simulink model "PWM_PI_PE_2018b"  (R2018b)
settings: Solver=VariableStepAuto  StartTime=0.0  StopTime=10e-3  RelTol=1e-3
values from neighbouring files (symbols this model uses):
  Ap = wc*Tr    (= 0.861890988639)    [PWM_szab_init.m]
  fs = 20e3    (= 20000)    [PWM_szab_init.m]
  k_peak = 10    [PWM_szab_init.m]
  Ki = xref_n/Iki_n    (= 1)    [PWM_szab_init.m]
  R = 0.1    [PWM_szab_init.m]
  tau_Ki = 2e-6    (= 2e-06)    [PWM_szab_init.m]
  TI = 1/(wc*tan((pi/2-fi_t)*1/3))    [PWM_szab_init.m]
undefined symbols (not defined in the file or in its folder): sigbuilder_block
libraries: ee_lib x8, nesl_utility x6, fl_lib x4, simulink x1
settings Model: Creator=kissd  LastModifiedBy=kissd
settings DataIOCC: ReturnWorkspaceOutputs=on

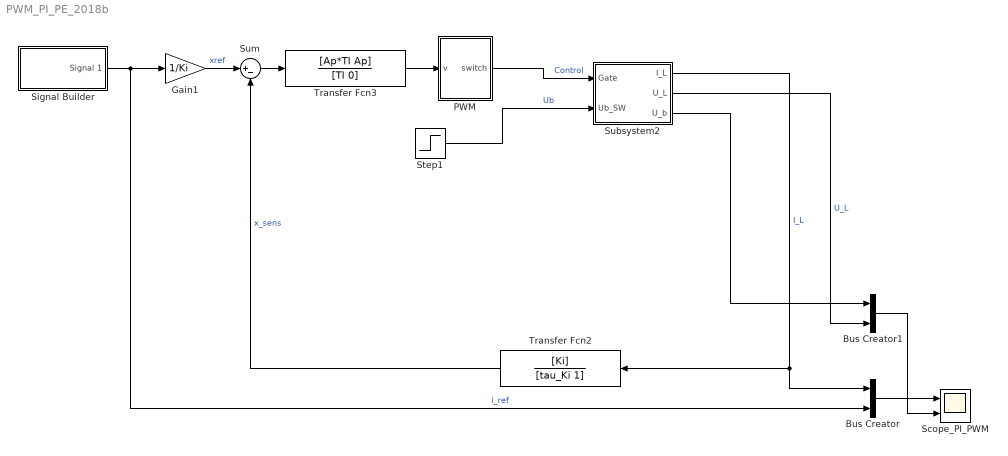
== system PWM_PI_PE_2018b ==
  Bus Creator : BusCreator  Inputs=2
  Bus Creator1 : BusCreator  Inputs=2
  Gain1 : Gain  Gain=1/Ki
  PWM : Subsystem
  Scope_PI_PWM : Scope  NumInputPorts=2
  Signal Builder : Subsystem  Tag=STV Subsys  LoadFcn=sigbuilder_block('load');  StartFcn=sigbuilder_block('start');  StopFcn=sigbuilder_block('stop');  ClipboardFcn=sigbuilder_block('clipboard');  mask(Sigbuilder block){tuvar=[0:10]}
      mask help: Simulink:masks:SigbuilderBlock_MD
      mask init:
      | if ~strcmp(get_param(bdroot(gcbh),'SimulationStatus'),'stopped') tuvar = sigbuilder_block('maskInit'); end
      settings: CopyFcn=sigbuilder_block('copy');  DeleteFcn=sigbuilder_block('delete');  ModelCloseFcn=sigbuilder_block('modelClose');  PreSaveFcn=sigbuilder_block('preSave');  PauseFcn=sigbuilder_block('pause');  ContinueFcn=sigbuilder_block('continue');  NameChangeFcn=sigbuilder_block('namechange');  OpenFcn=sigbuilder_block('open',[437.25 118.5 550.5 394.5 ]);  CloseFcn=sigbuilder_block('close');
      mask Display: plot(0, 0, 100, 100,[2, 2, 32, 32, 2], [68, 8, 8, 68, 68],[32, 2], [38, 38], [32, 19, 2],[53, 60, 44], [32, 17, 17, 2],[16, 16, 31, 31]);txt = getActiveGroup(gcbh);text(2, 100, txt,'verticalAlignment', 'top');
  Step1 : Step  Time=6e-3  SampleTime=0
  Subsystem2 : Subsystem
  Sum : Sum  Inputs=|+-
  Transfer Fcn2 : TransferFcn  Numerator=[Ki]  Denominator=[tau_Ki 1]
  Transfer Fcn3 : TransferFcn  Numerator=[Ap*TI Ap]  Denominator=[TI 0]
  wires:
  Transfer Fcn3/1 -> PWM/1(v)
  Signal Builder/1(Signal 1) -> Bus Creator/2, Gain1/1  "i_ref"
  Bus Creator/1 -> Scope_PI_PWM/1
  Bus Creator1/1 -> Scope_PI_PWM/2
  Transfer Fcn2/1 -> Sum/2  "x_sens"
  Subsystem2/2(U_L) -> Bus Creator1/2  "U_L"
  Gain1/1 -> Sum/1  "xref"
  PWM/1(switch) -> Subsystem2/1(Gate)  "Control"
  Subsystem2/1(I_L) -> Bus Creator/1, Transfer Fcn2/1  "I_L"
  Sum/1 -> Transfer Fcn3/1
  Step1/1 -> Subsystem2/2(Ub_SW)  "Ub"
  Subsystem2/3(U_b) -> Bus Creator1/1

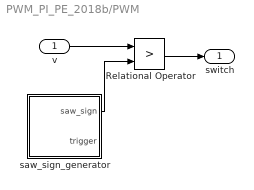
== system PWM_PI_PE_2018b/PWM ==
  v : Inport
  Relational Operator : RelationalOperator  Operator=>  OutDataTypeStr=boolean  ZeroCross=off  RndMeth=Nearest
  saw_sign_generator : Subsystem
  switch : Outport  VectorParamsAs1DForOutWhenUnconnected=off
  wires:
  Relational Operator/1 -> switch/1
  v/1 -> Relational Operator/1
  saw_sign_generator/1(saw_sign) -> Relational Operator/2

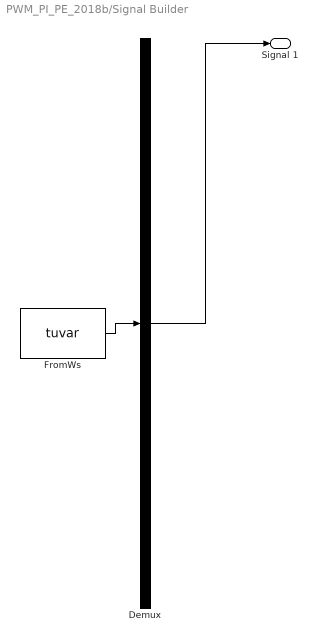
== system PWM_PI_PE_2018b/Signal Builder ==
  Demux : Demux  Tag=STV Demux  Outputs=1
  FromWs : FromWorkspace  Tag=STV FromWs  VariableName=tuvar  SampleTime=0
      SigBuilderData=|
      | common.afterFinalStr = 'Extrapolate'
      | common.sampleTime = 0
      | dataSet.timeRange = [0 10]
      | dataSet.name = 'Group 1'
      | sbobj.Groups.Name = 'Group 1'
      | sbobj.Groups.Signals.Name = 'Signal 1'
      | sbobj.Groups.Signals.XData = [0 0.0001 0.00011 6 6 10]
      | sbobj.Groups.Signals.YData = [0 0 10 10 0 0]
  Signal 1 : Outport  Tag=STV Outport  VectorParamsAs1DForOutWhenUnconnected=off
  wires:
  Demux/1 -> Signal 1/1
  FromWs/1 -> Demux/1

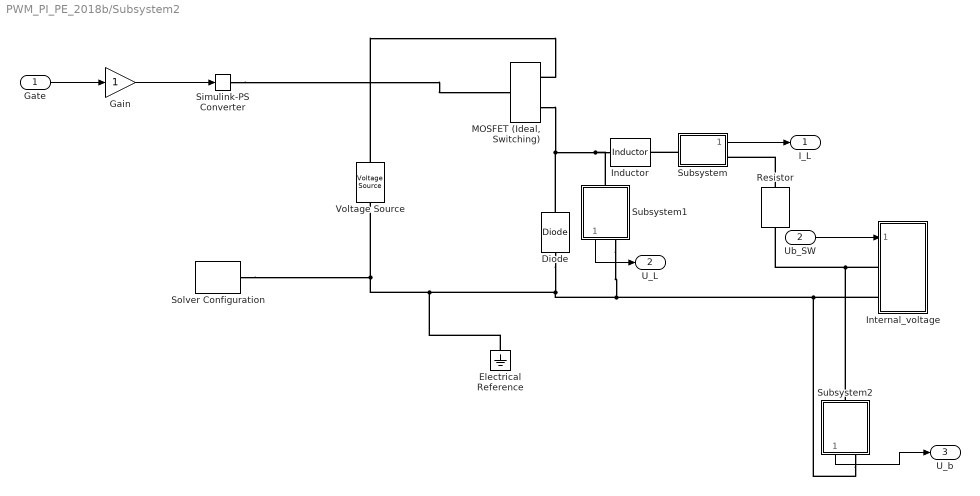
== system PWM_PI_PE_2018b/Subsystem2 ==
  Gate : Inport
  Ub_SW : Inport  Port=2
  Diode : ee_lib/Semiconductors & Converters/Diode  ModelType=ee.enum.diode.modelType.pwl  Vf=0.1 V  Ron=0.3 Ohm  Goff=1e-8 S  prmExp=ee.enum.diode.expParam.useTwo  I12=[.0137, .545] A  V12=[.6, .7] V  IS=1e-12 A  ec=1  I1=0.0137 A  V1=0.6 V  RS=0 Ohm  Tmeas=25 degC  N_series=1  N_parallel=1  Rz=0.3 Ohm  BV=inf V  C_param=ee.enum.diode.capParam.fixed  CJ=5 pF  CJ0=5 pF  VJ=1 V  Mgrad=0.5  Vvec=[.1, 10, 100] V  Cvec=[3.5, 1, .4] pF  FC=0.5  Q_param=ee.enum.diode.recoveryParam.off  iRM=-7.15 A  iF=4 A  didt=-750 A/us  trr_factor=3  trr=115 ns  Qrr=1500 s*uA  TT=50 ns  tau=100 ns  T_param=ee.enum.diode.temperatureParam.off  IS_T2=1.25e-7 A  I1_T2=0.245 A  V1_T2=0.5 V  Tmeas2=125 degC  EG_param=ee.enum.diode.egapParam.material_si  EG=1.11 eV  XTI_param=ee.enum.diode.xtiParam.pn  XTI=3  dBVdT=0 V/K  Tdevice=25 degC  i_specify=off  i_priority=None  i=0 A  i_nominal_specify=off  i_nominal_unit=A  i_nominal_value=1  v_specify=off  v_priority=None  v=0 V  v_nominal_specify=off  v_nominal_unit=V  v_nominal_value=1  i_capacitor_specify=off  i_capacitor_priority=None  i_capacitor=0 A  i_capacitor_nominal_specify=off  i_capacitor_nominal_unit=A  i_capacitor_nominal_value=1  v_capacitor_specify=off  v_capacitor_priority=None  v_capacitor=0 V  v_capacitor_nominal_specify=off  v_capacitor_nominal_unit=V  v_capacitor_nominal_value=1  power_dissipated_specify=off  power_dissipated_priority=None  power_dissipated=0 W  power_dissipated_nominal_specify=off  power_dissipated_nominal_unit=W  power_dissipated_nominal_value=1  thermal_network_parameterization=ee.enum.thermalNetworkTopology.cauer  Rth=[0, 10] K/W  Rth_Foster=[4, 6] K/W  thermal_mass_parameterization=ee.enum.thermalNetwork.timeconstant  thermal_mass=[0, 1] J/K  thermal_mass_Foster=[1.5, 3] J/K  thermal_time_constant=[0, 10] s  thermal_time_constant_Foster=[6, 18] s  thermal_mass_initial_temperatures=[25, 25] degC
      settings: SourceProductName=Simscape Electrical
  Electrical Reference : fl_lib/Electrical/Electrical Elements/Electrical Reference
  Gain : Gain  OutDataTypeStr=double
  Inductor : ee_lib/Passive/Inductor  l=L H  L_tol=20  enable_L_tol=0  tol_distribution=1  nSigma=4  r=0 Ohm  g=1e-9 1/Ohm  enable_operating_limits=0  operating_limit_action=2  max_working_current=1 A  power_rating=1 W  enable_faults=0  fault_action=1  lambdaPercent=50  k_faulted=0.9999  turnsShort=0  openCct=0  groundShort=0  groundShortG=0 1/Ohm  tau_fault=1e-3 s  enable_temporal_fault=0  t_fault=1 s  enable_behavioral_fault=0  max_permissible_voltage=100 V  n_fail_on_voltage=1  max_permissible_current=1 A  t_fail_on_current=1 s  i_L_specify=off  i_L_priority=High  i_L=0 A  i_L_nominal_specify=off  i_L_nominal_unit=A  i_L_nominal_value=1
      settings: SourceProductName=Simscape Electrical
  Internal_voltage : Subsystem
  "MOSFET (Ideal, Switching)" : ee_lib/Semiconductors & Converters/MOSFET (Ideal, Switching)  Rds=0.001 Ohm  Goff=1e-6 1/Ohm  Vth=0.8 V  diode_param=1  diode_Vf=0.8 V  diode_Ron=0.001 Ohm  diode_Goff=1e-5 1/Ohm  diode_C=50e-9 F  diode_iRM=-235 A  diode_iF=300 A  diode_idot=-50 A/us  diode_trr_param=1  diode_trr_factor=3  diode_trr=15 us  diode_Qrr=1500 s*uA  thermal_loss_option=2  Voff=300 V  Tau=1e-4 s  Tj=[298.15, 398.15] K  Iout_scalar=600 A  Eon_scalar=22.86e-3 J  Eoff_scalar=17.14e-3 J  Von_scalar=2.7 V  Iout_data=[0, 10, 50, 100, 200, 400, 600] A  Eon_data=[0, .29, 1.43, 2.86, 5.71, 13.14, 22.86; 0, .57, 2.63, 5.14, 10.29, 20.57, 30.29] * 1e-3 J  Eoff_data=[0, .21, 1.07, 2.14, 4.29, 9.86, 17.14; 0, .43, 1.97, 3.86, 7.71, 15.43, 22.71] * 1e-3 J  Von_data=[0, 1.1, 1.3, 1.45, 1.75, 2.25, 2.7; 0, 1, 1.15, 1.35, 1.7, 2.35, 3] V
      settings: SourceProductName=Simscape Electrical
  Resistor : ee_lib/Passive/Resistor  R=R Ohm  R_tol=5  enable_R_tol=0  tol_distribution=1  nSigma=4  enable_operating_limits=0  operating_limit_action=2  max_working_voltage=100 V  power_rating=1 W  enable_faults=0  fault_action=1  R_faulted=inf Ohm  enable_temporal_fault=0  t_fault=1 s  enable_behavioral_fault=0  max_permissible_current=1 A  t_fail_on_current=1 s  noise_mode=0  sample_time=1e-3 s  repeatability=1  auto_seed=1852908280  user_seed=0  Tdevice=25 degC  alpha=3.93e-3 1/K  Tmeas=25 degC  thermal_mass=100 J/K  power_derating_T1=70 degC  power_derating_T2=155 degC  operating_temperature_range_vec=[-50, 150] degC  temperature_specify=off  temperature_priority=High  temperature=298.15 K  temperature_nominal_specify=off  temperature_nominal_unit=K  temperature_nominal_value=1
      settings: SourceProductName=Simscape Electrical
  Simulink-PS Converter : nesl_utility/Simulink-PS Converter  PhysicalDomain=network_engine_domain  SubClassName=ps_input  LeftPortType=input  RightPortType=output  PseudoPeriodic=off  Frequencies=[]  NoiseDistribution=none  NoiseParameters=[]  Unit=1  AffineConversion=off  FilteringAndDerivatives=provide  SimscapeFilterOrder=1  InputFilterTimeConstant=0.001  UdotUserProvided=0
  Solver Configuration : nesl_utility/Solver Configuration  PhysicalDomain=network_engine_domain  SubClassName=solver  LeftPortType=input  RightPortType=generic  Tones=[]  Harmonics=[]  SimulateNoise=off  Profile=off  UseLocalSampling=off  EnableSwitchedLinearOptims=on  FrequencyDomain=off  UseCCode=off  RelTol=0.001  AbsTol=1e-06  MinStep=1e-09  ToWorkspace=off  RevertToSquareIcSolve=off  NumHomotopyIterations=100  PhasorMode=off  PhasorModeNumHarmonics=1  DoDC=off  ResidualTolerance=1e-09  UseLocalSolver=on  LocalSolverChoice=NE_BACKWARD_EULER_ADVANCER  LocalSolverSampleTime=1e-7  DoFixedCost=on  MaxNonlinIter=3  MaxModeIter=2  LinearAlgebra=auto  EquationFormulation=NE_TIME_EF  DelaysMemoryBudget=1024  AutomaticFiltering=on  FilteringTimeConstant=0.001  PartitionStorageMethod=AS_NEEDED  PartitionMemoryBudget=1024  PartitionMethod=ROBUST
  Subsystem : Subsystem
  Subsystem1 : Subsystem
  Subsystem2 : Subsystem
  Voltage Source : ee_lib/Sources/Voltage Source  dc_voltage=U_dc V  ac_voltage=0 V  ac_shift=0 rad  ac_frequency=60 Hz  noise_mode=0  PSD=0 V^2/Hz  repeatability=1  auto_seed=3499211588  user_seed=0  sample_time=1e-3 s  i_specify=off  i_priority=None  i=0 A  i_nominal_specify=off  i_nominal_unit=A  i_nominal_value=1  v_specify=off  v_priority=None  v=0 V  v_nominal_specify=off  v_nominal_unit=V  v_nominal_value=1
      settings: SourceProductName=Simscape Electrical
  I_L : Outport
  U_L : Outport  Port=2
  U_b : Outport  Port=3
  wires:
  Subsystem/1(I_signal) -> I_L/1
  Gate/1 -> Gain/1
  Subsystem1/1(V_signal) -> U_L/1
  Ub_SW/1 -> Internal_voltage/1(Control)
  Gain/1 -> Simulink-PS Converter/1
  Subsystem2/1(V_signal) -> U_b/1
  connections:
  Electrical Reference/LConn1 -- Solver Configuration/RConn1 -- Voltage Source/RConn1 -- Diode/LConn1 -- Subsystem2/RConn1 -- Internal_voltage/LConn2 -- Subsystem1/RConn1
  Resistor/LConn1 -- Subsystem/RConn1
  Simulink-PS Converter/RConn1 -- "MOSFET (Ideal, Switching)"/LConn1
  Internal_voltage/LConn1 -- Resistor/RConn1 -- Subsystem2/LConn1
  "MOSFET (Ideal, Switching)"/RConn2 -- Diode/RConn1 -- Subsystem1/LConn1 -- Inductor/LConn1
  Subsystem/LConn1 -- Inductor/RConn1
  Voltage Source/LConn1 -- "MOSFET (Ideal, Switching)"/RConn1

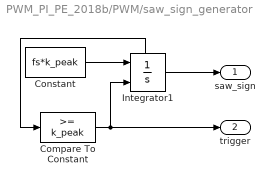
== system PWM_PI_PE_2018b/PWM/saw_sign_generator ==
  Compare To Constant : simulink/Logic and Bit Operations/Compare To Constant  relop=>=  const=k_peak  OutDataTypeStr=boolean
  Constant : Constant  Value=fs*k_peak
  Integrator1 : Integrator  ExternalReset=rising  ShowStatePort=on
  saw_sign : Outport  VectorParamsAs1DForOutWhenUnconnected=off
  trigger : Outport  Port=2  VectorParamsAs1DForOutWhenUnconnected=off
  wires:
  Integrator1/1 -> saw_sign/1
  Integrator1/State -> Compare To Constant/1
  Constant/1 -> Integrator1/1
  Compare To Constant/1 -> trigger/1, Integrator1/2

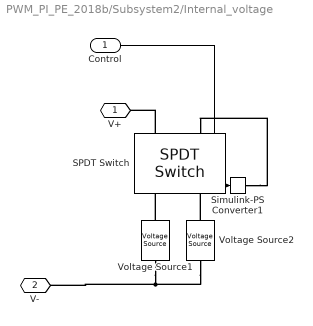
== system PWM_PI_PE_2018b/Subsystem2/Internal_voltage ==
  Control : Inport
  SPDT Switch : ee_lib/Switches & Breakers/SPDT Switch  R_closed=0.001 Ohm  G_open=1e-6 S  Threshold=0.5 V  Width=0 V  model_dynamics=0  t_on=1e-3 s  t_off=1e-3 s  initial_vT=0 V
      settings: SourceProductName=Simscape Electrical  SourceProductBaseCode=PS
  Simulink-PS Converter1 : nesl_utility/Simulink-PS Converter  PhysicalDomain=network_engine_domain  SubClassName=ps_input  LeftPortType=input  RightPortType=output  PseudoPeriodic=off  Frequencies=[]  NoiseDistribution=none  NoiseParameters=[]  Unit=1  AffineConversion=off  FilteringAndDerivatives=provide  SimscapeFilterOrder=1  InputFilterTimeConstant=0.001  UdotUserProvided=0
  Voltage Source1 : ee_lib/Sources/Voltage Source  dc_voltage=70 V  ac_voltage=0 V  ac_shift=0 rad  ac_frequency=60 Hz  noise_mode=0  PSD=0 V^2/Hz  repeatability=1  auto_seed=4059491904  user_seed=0  sample_time=1e-3 s  i_specify=off  i_priority=None  i=0 A  i_nominal_specify=off  i_nominal_unit=A  i_nominal_value=1  v_specify=off  v_priority=None  v=0 V  v_nominal_specify=off  v_nominal_unit=V  v_nominal_value=1
      settings: SourceProductName=Simscape Electrical
  Voltage Source2 : ee_lib/Sources/Voltage Source  dc_voltage=20 V  ac_voltage=0 V  ac_shift=0 rad  ac_frequency=60 Hz  noise_mode=0  PSD=0 V^2/Hz  repeatability=1  auto_seed=2256594732  user_seed=0  sample_time=1e-3 s  i_specify=off  i_priority=None  i=0 A  i_nominal_specify=off  i_nominal_unit=A  i_nominal_value=1  v_specify=off  v_priority=None  v=0 V  v_nominal_specify=off  v_nominal_unit=V  v_nominal_value=1
      settings: SourceProductName=Simscape Electrical
  V+ : PMIOPort  Side=Left
  V- : PMIOPort  Port=2  Side=Left
  wires:
  Control/1 -> Simulink-PS Converter1/1
  connections:
  Voltage Source1/LConn1 -- SPDT Switch/RConn2
  Voltage Source2/LConn1 -- SPDT Switch/RConn1
  SPDT Switch/LConn2 -- V+/RConn1
  Simulink-PS Converter1/RConn1 -- SPDT Switch/LConn1
  Voltage Source1/RConn1 -- V-/RConn1 -- Voltage Source2/RConn1

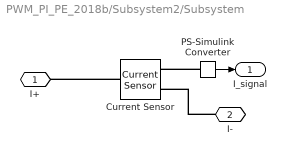
== system PWM_PI_PE_2018b/Subsystem2/Subsystem ==
  Current Sensor : fl_lib/Electrical/Electrical Sensors/Current Sensor
  PS-Simulink Converter : nesl_utility/PS-Simulink Converter  PhysicalDomain=network_engine_domain  SubClassName=ps_output  LeftPortType=input  RightPortType=output  PseudoPeriodic=off  Frequencies=[]  Unit=inherit  AffineConversion=off
  I+ : PMIOPort  Side=Left
  I- : PMIOPort  Port=2  Side=Right
  I_signal : Outport
  wires:
  PS-Simulink Converter/1 -> I_signal/1
  connections:
  PS-Simulink Converter/LConn1 -- Current Sensor/RConn1
  Current Sensor/LConn1 -- I+/RConn1
  I-/RConn1 -- Current Sensor/RConn2

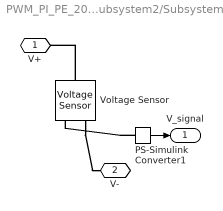
== system PWM_PI_PE_2018b/Subsystem2/Subsystem1 ==
  PS-Simulink Converter1 : nesl_utility/PS-Simulink Converter  PhysicalDomain=network_engine_domain  SubClassName=ps_output  LeftPortType=input  RightPortType=output  PseudoPeriodic=off  Frequencies=[]  Unit=inherit  AffineConversion=off
  Voltage Sensor : fl_lib/Electrical/Electrical Sensors/Voltage Sensor
  V+ : PMIOPort  Side=Left
  V- : PMIOPort  Port=2  Side=Right
  V_signal : Outport
  wires:
  PS-Simulink Converter1/1 -> V_signal/1
  connections:
  Voltage Sensor/RConn2 -- V-/RConn1
  PS-Simulink Converter1/LConn1 -- Voltage Sensor/RConn1
  Voltage Sensor/LConn1 -- V+/RConn1

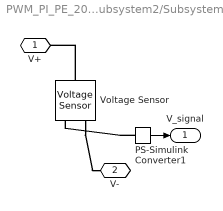
== system PWM_PI_PE_2018b/Subsystem2/Subsystem2 ==
  PS-Simulink Converter1 : nesl_utility/PS-Simulink Converter  PhysicalDomain=network_engine_domain  SubClassName=ps_output  LeftPortType=input  RightPortType=output  PseudoPeriodic=off  Frequencies=[]  Unit=inherit  AffineConversion=off
  Voltage Sensor : fl_lib/Electrical/Electrical Sensors/Voltage Sensor
  V+ : PMIOPort  Side=Left
  V- : PMIOPort  Port=2  Side=Right
  V_signal : Outport
  wires:
  PS-Simulink Converter1/1 -> V_signal/1
  connections:
  Voltage Sensor/RConn2 -- V-/RConn1
  PS-Simulink Converter1/LConn1 -- Voltage Sensor/RConn1
  Voltage Sensor/LConn1 -- V+/RConn1
